simulink subsystem "Orient_update"  (R2025b)
settings: Solver=VariableStepAuto  StartTime=0.0  StopTime=10.0  RelTol=1e-3
settings Model: Creator=Admin  LastModifiedBy=Admin

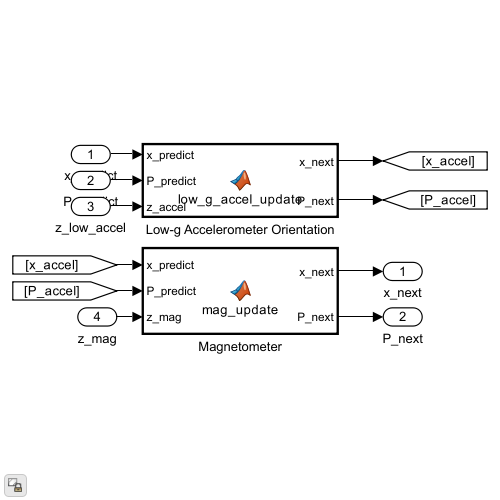
[thumbnail: Simulink's stored preview of the top-level diagram]
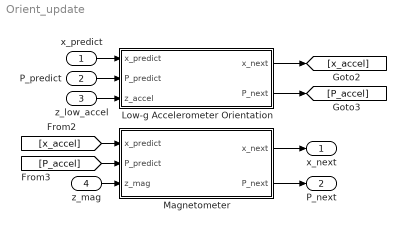
== system Orient_update ==
  x_predict : Inport
  P_predict : Inport  Port=2
  z_low_accel : Inport  Port=3
  z_mag : Inport  Port=4
  Low-g Accelerometer Orientation : MATLAB Function  TreatAsAtomicUnit=on
  Magnetometer : MATLAB Function  TreatAsAtomicUnit=on
  x_next : Outport
  P_next : Outport  Port=2
  wires:
  Low-g Accelerometer Orientation/1(x_next) -> [x_accel]
  [x_accel] -> Magnetometer/1(x_predict)
  [P_accel] -> Magnetometer/2(P_predict)
  z_mag/1 -> Magnetometer/3(z_mag)
  Low-g Accelerometer Orientation/2(P_next) -> [P_accel]
  Magnetometer/2(P_next) -> P_next/1
  Magnetometer/1(x_next) -> x_next/1
  x_predict/1 -> Low-g Accelerometer Orientation/1(x_predict)
  P_predict/1 -> Low-g Accelerometer Orientation/2(P_predict)
  z_low_accel/1 -> Low-g Accelerometer Orientation/3(z_accel)

== matlab function Orient_update/Magnetometer ==
  data: x_predict input; x_next output; P_predict input; z_mag input; P_next output
function [x_next, P_next] = mag_update(x_predict, P_predict, z_mag)
%MAG_UPDATE Magnetometer measurement update
%
% x = [p(3); v(3); q(4); bg(3); ba_high(3); ba_low(3)]   -> 19 states
%
% z_mag(1:3) = measured magnetic field in body frame
% z_mag(4:6) = reference magnetic field in NED frame

sigma_mag = 0.05;
R = (sigma_mag^2) * eye(3);
n = 19;

m_n    = z_mag(4:6);
z_meas = z_mag(1:3);

% Guard against zero vectors on both
if norm(z_meas) < 1e-9 || norm(m_n) < 1e-9
    x_next = x_predict;
    P_next = P_predict;
    return;
end

% Normalise
z_meas = z_meas / norm(z_meas);
m_n    = m_n    / norm(m_n);

mN = m_n(1);
mE = m_n(2);
mD = m_n(3);

% Extract and normalise quaternion [w x y z]
q = x_predict(7:10);
if norm(q) < 1e-9
    q = [1;0;0;0];
else
    q = q / norm(q);
end
q0 = q(1); q1 = q(2); q2 = q(3); q3 = q(4);

% Predicted body-frame measurement via explicit DCM (NED -> body)
h = ned2body(m_n, q);

% Analytic Jacobian dh/dq (3x4)
Hq = [ ...
     2*q3*mE - 2*q2*mD,           2*q2*mE + 2*q3*mD,           -4*q2*mN + 2*q1*mE - 2*q0*mD,  -4*q3*mN + 2*q0*mE + 2*q1*mD; ...
    -2*q3*mN + 2*q1*mD,           2*q2*mN - 4*q1*mE + 2*q0*mD,  2*q1*mN + 2*q3*mD,            -2*q0*mN - 4*q3*mE + 2*q2*mD; ...
     2*q2*mN - 2*q1*mE,           2*q3*mN - 2*q0*mE - 4*q1*mD,  2*q0*mN + 2*q3*mE - 4*q2*mD,  2*q1*mN + 2*q2*mE           ];

% Tangent-space projection — keeps correction orthogonal to q
Hq = Hq * (eye(4) - q * q');

% Full 3x19 measurement Jacobian
H = [zeros(3,6), Hq, zeros(3,9)];

% Kalman gain
S   = H * P_predict * H' + R;
K_k = P_predict * H' / S;

% State update
x_next = x_predict + K_k * (z_meas - h);

% Joseph-form covariance update (numerically stable)
IKH    = eye(n) - K_k * H;
P_next = IKH * P_predict * IKH' + K_k * R * K_k';

% Enforce symmetry to prevent numerical drift in P
P_next = (P_next + P_next') / 2;

% Renormalise quaternion
q_new = x_next(7:10);
if norm(q_new) < 1e-9
    x_next(7:10) = [1;0;0;0];
else
    x_next(7:10) = q_new / norm(q_new);
end

end

== matlab function Orient_update/Low-g Accelerometer Orientation ==
  data: x_predict input; x_next output; P_predict input; z_accel input; P_next output
function [x_next, P_next] = low_g_accel_update(x_predict, P_predict, z_accel)
%LOW_G_ACCEL_UPDATE  EKF measurement update — accelerometer gravity alignment
%  Orientation-only update: corrects q and ba_low.
%  Valid only when sensor is near-static (|a| ≈ g).
%
%  State:  x = [p(3); v(3); q(4); bg(3); ba_high(3); ba_low(3)]  (19x1)
%   p  : 1:3    v  : 4:6    q  : 7:10
%   bg : 11:13  ba_high : 14:16  ba_low : 17:19

g = 9.81;
n = 19;

%% ── Guards ───────────────────────────────────────────────────────────────────
z_accel  = z_accel(:);
z_norm   = norm(z_accel);

if ~isfinite(z_norm) || z_norm < 1e-9
    x_next = x_predict;  P_next = P_predict;  return
end

if abs(z_norm - g) > 2.0          % not near-static — skip update
    x_next = x_predict;  P_next = P_predict;  return
end

%% ── Extract states ───────────────────────────────────────────────────────────
q      = x_predict(7:10);
ba_low = x_predict(17:19);

q_norm = norm(q);
if ~isfinite(q_norm) || q_norm < 1e-9
    q = [1;0;0;0];
else
    q = q / q_norm;
end
q0=q(1); q1=q(2); q2=q(3); q3=q(4);

%% ── Measurement model ────────────────────────────────────────────────────────
% Static specific force in body frame = ned2body(-g_ned) + bias
h = ned2body([0;0;-g], q) + ba_low;

%% ── Jacobian ∂h/∂q  [3×4] ───────────────────────────────────────────────────
% h_no_bias = R_bn * [0;0;-g]  where R_bn is NED-to-body
% h1 = -g * 2(q1*q3 - q0*q2)
% h2 = -g * 2(q2*q3 + q0*q1)
% h3 = -g * (1 - 2*q1^2 - 2*q2^2)
Hq = 9.81 * [ 2*q2,  -2*q3,   2*q0,  -2*q1;
             -2*q1,  -2*q0,  -2*q3,  -2*q2;
             -2*q0,   2*q1,   2*q2,  -2*q3];

%% ── Full H [3×19] ────────────────────────────────────────────────────────────
%  Only q (cols 7:10) and ba_low (cols 17:19) are observed
H = zeros(3, 19);
H(:, 7:10)  = Hq;
H(:, 17:19) = eye(3);

%% ── Kalman gain ──────────────────────────────────────────────────────────────
sigma_accel = 0.005;
R_meas = (sigma_accel^2) * eye(3);

S = H * P_predict * H' + R_meas;
K = P_predict * H' / S;            % 19×3

%% ── Orientation-only: zero K rows for states we don't update ─────────────────
K(1:6,   :) = 0;     % p, v
K(11:16, :) = 0;     % bg, ba_high

%% ── State update ─────────────────────────────────────────────────────────────
x_next = x_predict + K * (z_accel - h);

%% ── Joseph-form covariance update ────────────────────────────────────────────
I19    = eye(n);
IKH    = I19 - K * H;
P_next = IKH * P_predict * IKH' + K * R_meas * K';
P_next = 0.5 * (P_next + P_next');

%% ── Renormalise quaternion ───────────────────────────────────────────────────
q_next = x_next(7:10);
q_norm = norm(q_next);
if ~isfinite(q_norm) || q_norm < 1e-9
    x_next(7:10) = [1;0;0;0];
else
    x_next(7:10) = q_next / q_norm;
end

end
